simulink model "RCAMSimulation"  (R2024a)
settings: Solver=VariableStepAuto  StartTime=0.0  StopTime=300  RelTol=1e-3
values from neighbouring files (symbols this model uses):
  dt = 1/50    (= 0.02)    [InitializeConstants.m]
  h0 = 250    [InitializeConstants.m]    (also in getDensityParams.m = 0)
  lat0 = deg2rad(47.608013)    [InitializeConstants.m]
  lon0 = deg2rad(-122.335167)    [InitializeConstants.m]
  u0_1 = [-6.32224925618250e-08 ... (first row only)    [InitializeConstants.m]
  u0_2 = [-6.32224925618250e-08 ... (first row only)    [InitializeConstants.m]
  x0 = [227.561443788829 ... (first row only)    [InitializeConstants.m]
undefined symbols (not defined in the file or in its folder): RCAM_Model
libraries: aerolibfltsims x2, matrix_library x1, aerolibanimutils x1
settings Model: Creator=athil  LastModifiedBy=athil
settings OptimizationCC: ReuseModelBlockBuffer=off
settings DebuggingCC: UnconnectedInputMsg=warning  UnconnectedOutputMsg=warning  UnconnectedLineMsg=warning
settings ModelReferenceCC: EnableRefExpFcnMdlSchedulingChecks=on
settings RTWCC: GPUComputeCapability=3.5  DLArmComputeVersion=19.05

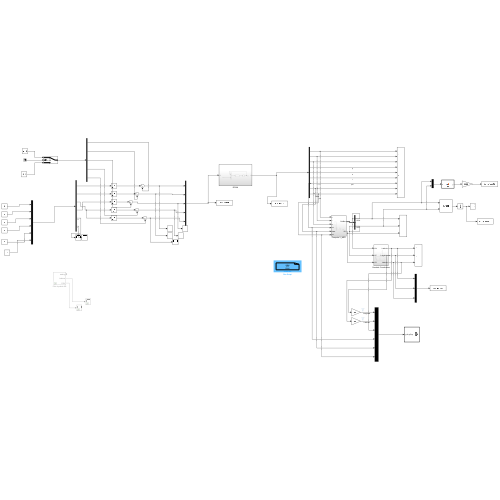
[thumbnail: Simulink's stored preview of the top-level diagram]
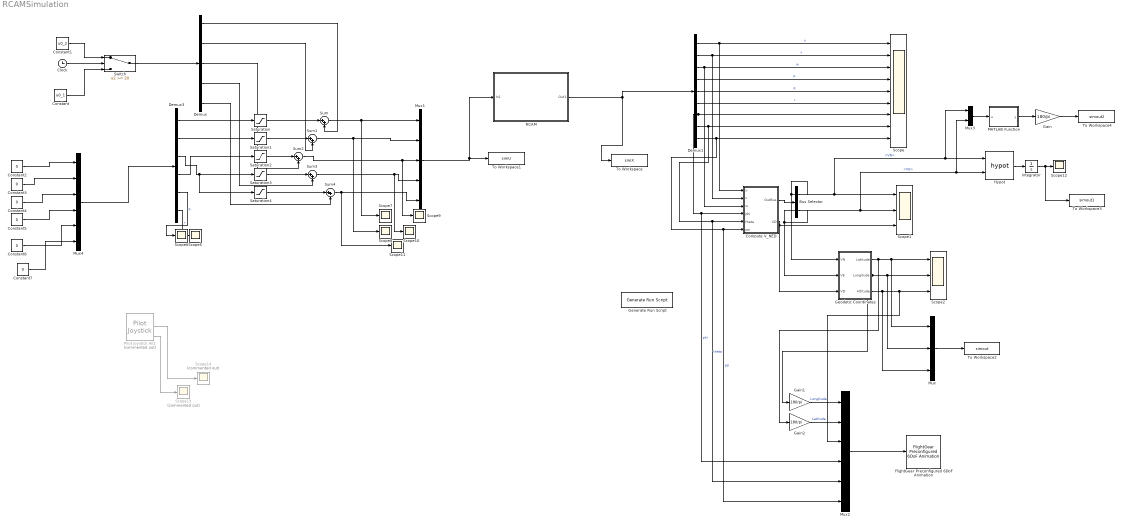
== system RCAMSimulation ==
  Bus Selector : BusSelector  OutputSignals=VN,VE
  Clock : Clock
  Compute V_NED : Subsystem
  Constant : Constant  Value=u0_1
  Constant1 : Constant  Value=u0_2
  Constant{2..7} (6 alike) : Constant  Value=0
  Demux : Demux  Outputs=5
  Demux1 : Demux  Outputs=9
  Demux3 : Demux  Outputs=6
  FlightGear Preconfigured 6DoF Animation : aerolibfltsims/FlightGear Preconfigured 6DoF Animation  xFlightGearVersion=v2019.1  DestinationIpAddress=127.0.0.1  DestinationPort=5502  SampleTime=1/50  packetVersion=24
  Gain : Gain  Gain=180/pi
  Gain1 : Gain  Gain=180/pi
  Gain2 : Gain  Gain=180/pi
  Generate Run Script : aerolibfltsims/Generate Run Script  Architecture=Default  dataFlow=Send  GeometryModelName=767-300  AirportId=KSFO  RunwayId=10L  InitialAltitude=7224  InitialHeading=113  OffsetDistance=4.72  OffsetAzimuth=0  InstallScenery=off  DisableShaders=on  OriginAddress=127.0.0.1  DestinationPort=5502  OriginPort=5505  LocalAddress=127.0.0.1  OutputFileName=runfg.bat  FlightGearBaseDirectory=C:\Program Files\FlightGear 2020.3
  Geodetic Coordinates : Subsystem
  Hypot : Math  Operator=hypot
  Integrator : Integrator
  MATLAB Function : MATLAB Function  TreatAsAtomicUnit=on
  Mux : Mux  Inputs=3
  Mux1 : Mux  Inputs=5
  Mux2 : Mux  Inputs=6
  Mux3 : Mux  Inputs=2
  Mux4 : Mux  Inputs=6
  Pilot Joystick All2 : aerolibanimutils/Pilot Joystick  Commented=on  JoystickID=Joystick1  OutputConfiguration=AllOutputs  SampleTime=dt
  RCAM : Subsystem
  Saturation{,1..4} (5 alike) : Saturate  UpperLimit=0.1  LowerLimit=-0.1
  Scope : Scope  NumInputPorts=9
  Scope1 : Scope  NumInputPorts=3
  Scope{5..12} (8 alike) : Scope
  Scope13 : Scope  Commented=on
  Scope14 : Scope  Commented=on
  Scope2 : Scope  NumInputPorts=3
  Sum{,1..4} (5 alike) : Sum  Inputs=|++
  Switch : Switch  Threshold=20  SaturateOnIntegerOverflow=off  InputSameDT=off
  To Workspace : ToWorkspace  VariableName=simX  SaveFormat=Timeseries  SampleTime=-1
  To Workspace1 : ToWorkspace  VariableName=simU  SaveFormat=Timeseries  SampleTime=-1
  To Workspace2 : ToWorkspace  VariableName=simout  SaveFormat=Timeseries  SampleTime=-1
  To Workspace3 : ToWorkspace  VariableName=simout1  SaveFormat=Timeseries  SampleTime=-1
  To Workspace4 : ToWorkspace  VariableName=simout2  SaveFormat=Timeseries  SampleTime=-1
  wires:
  Demux3/1 -> Saturation/1
  Demux3/2 -> Saturation1/1
  Saturation/1 -> Sum/1
  Mux1/1 -> RCAM/1(In1), To Workspace1/1
  Demux1/1 -> Scope/1, Compute V_NED/1(u)  "u"
  Demux1/3 -> Scope/3, Compute V_NED/3(w)  "w"
  Demux1/4 -> Scope/4  "p"
  Demux1/5 -> Scope/5  "q"
  Demux1/6 -> Scope/6  "r"
  Demux1/7 -> Scope/7, Mux2/4, Compute V_NED/4(phi)  "phi"
  Demux1/8 -> Scope/8, Mux2/5, Compute V_NED/5(theta)  "theta"
  Demux1/9 -> Scope/9, Mux2/6, Compute V_NED/6(psi)  "psi"
  Demux1/2 -> Scope/2, Compute V_NED/2(v)  "v"
  Bus Selector/1 -> Mux3/1, Hypot/1, Scope1/1, Geodetic Coordinates/1(VN)  "<VN>"
  Bus Selector/2 -> Mux3/2, Hypot/2, Scope1/2, Geodetic Coordinates/2(VE)  "<VE>"
  Compute V_NED/2(VD) -> Geodetic Coordinates/3(VD), Scope1/3
  Geodetic Coordinates/1(Latitude) -> Gain2/1, Mux/1, Scope2/1
  Geodetic Coordinates/2(Longitude) -> Gain1/1, Mux/2, Scope2/2
  Mux2/1 -> FlightGear Preconfigured 6DoF Animation/1
  Gain1/1 -> Mux2/1  "Longitude"
  Gain2/1 -> Mux2/2  "Latitude"
  Geodetic Coordinates/3(Altitude) -> Mux/3, Mux2/3, Scope2/3
  RCAM/1(Out1) -> Demux1/1, To Workspace/1
  Demux3/5 -> Scope6/1  "q"
  Demux3/6 -> Scope5/1  "r"
  Mux/1 -> To Workspace2/1
  Compute V_NED/1(OutBus) -> Bus Selector/1
  Demux/1 -> Sum/2
  Sum/1 -> Scope7/1, Mux1/1
  Saturation1/1 -> Sum1/1
  Demux/2 -> Sum1/2
  Sum1/1 -> Scope8/1, Mux1/2
  Saturation2/1 -> Sum2/1
  Demux/3 -> Sum2/2
  Sum2/1 -> Scope9/1, Mux1/3
  Saturation3/1 -> Sum3/1
  Demux/4 -> Sum3/2
  Sum3/1 -> Scope10/1, Mux1/4
  Saturation4/1 -> Sum4/1
  Demux/5 -> Sum4/2
  Sum4/1 -> Scope11/1, Mux1/5
  Demux3/4 -> Saturation2/1
  Demux3/3 -> Saturation4/1, Saturation3/1
  Hypot/1 -> Integrator/1
  Integrator/1 -> To Workspace3/1, Scope12/1
  Mux3/1 -> MATLAB Function/1(u)
  MATLAB Function/1(y) -> Gain/1
  Gain/1 -> To Workspace4/1
  Clock/1 -> Switch/2
  Switch/1 -> Demux/1
  Constant1/1 -> Switch/1
  Constant/1 -> Switch/3
  Pilot Joystick All2/2 -> Scope14/1
  Pilot Joystick All2/3 -> Scope13/1
  Constant2/1 -> Mux4/1
  Constant3/1 -> Mux4/2
  Constant4/1 -> Mux4/3
  Constant5/1 -> Mux4/4
  Constant6/1 -> Mux4/5
  Constant7/1 -> Mux4/6
  Mux4/1 -> Demux3/1

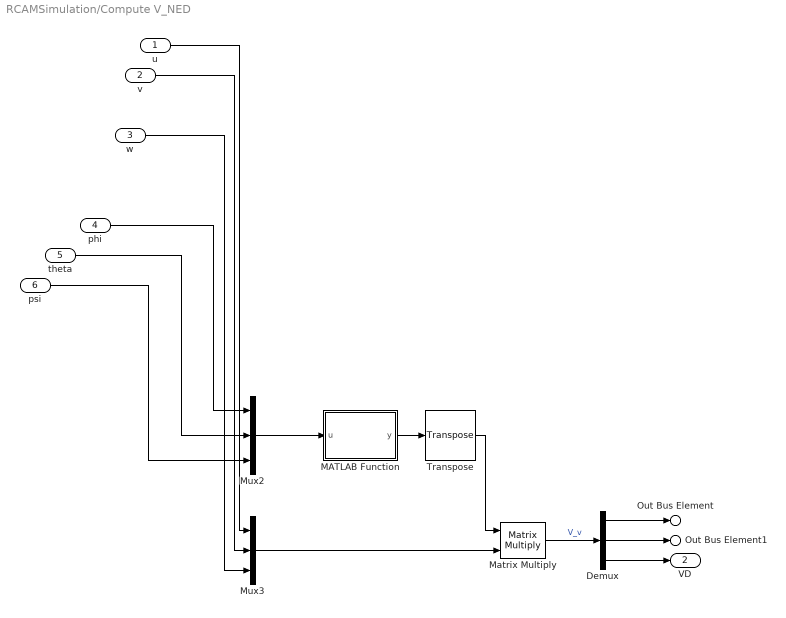
== system RCAMSimulation/Compute V_NED ==
  u : Inport
  v : Inport  Port=2
  w : Inport  Port=3
  phi : Inport  Port=4
  theta : Inport  Port=5
  psi : Inport  Port=6
  Demux : Demux  Outputs=3
  MATLAB Function : MATLAB Function  TreatAsAtomicUnit=on
  Matrix Multiply : Product  Multiplication=Matrix(*)
  Mux2 : Mux  Inputs=3
  Mux3 : Mux  Inputs=3
  Transpose : matrix_library/Transpose
  Out Bus Element : Outport  PortName=OutBus  Element=VN
  Out Bus Element1 : Outport  PortName=OutBus  Element=VE
  VD : Outport  Port=2
  wires:
  MATLAB Function/1(y) -> Transpose/1
  phi/1 -> Mux2/1
  Mux3/1 -> Matrix Multiply/2
  Mux2/1 -> MATLAB Function/1(u)
  Transpose/1 -> Matrix Multiply/1
  v/1 -> Mux3/2
  theta/1 -> Mux2/2
  w/1 -> Mux3/3
  psi/1 -> Mux2/3
  u/1 -> Mux3/1
  Matrix Multiply/1 -> Demux/1  "V_v"
  Demux/1 -> Out Bus Element/1
  Demux/2 -> Out Bus Element1/1
  Demux/3 -> VD/1

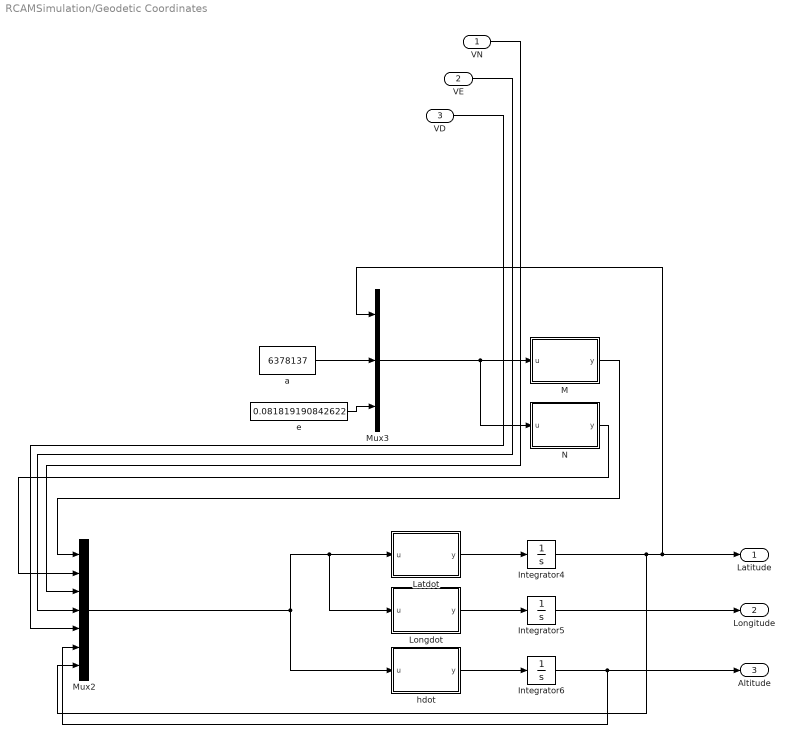
== system RCAMSimulation/Geodetic Coordinates ==
  VN : Inport
  VE : Inport  Port=2
  VD : Inport  Port=3
  Integrator4 : Integrator  InitialCondition=lat0
  Integrator5 : Integrator  InitialCondition=lon0
  Integrator6 : Integrator  InitialCondition=h0
  Latdot : MATLAB Function  TreatAsAtomicUnit=on
  Longdot : MATLAB Function  TreatAsAtomicUnit=on
  M : MATLAB Function  TreatAsAtomicUnit=on
  Mux2 : Mux  Inputs=7
  Mux3 : Mux  Inputs=3
  N : MATLAB Function  TreatAsAtomicUnit=on
  a : Constant  Value=6378137
  e : Constant  Value=0.081819190842622
  hdot : MATLAB Function  TreatAsAtomicUnit=on
  Latitude : Outport
  Longitude : Outport  Port=2
  Altitude : Outport  Port=3
  wires:
  VE/1 -> Mux2/4
  M/1(y) -> Mux2/1
  Integrator6/1 -> Altitude/1, Mux2/6
  hdot/1(y) -> Integrator6/1
  Mux2/1 -> Longdot/1(u), Latdot/1(u), hdot/1(u)
  Mux3/1 -> N/1(u), M/1(u)
  N/1(y) -> Mux2/2
  a/1 -> Mux3/2
  Integrator4/1 -> Mux2/7, Latitude/1, Mux3/1
  e/1 -> Mux3/3
  Latdot/1(y) -> Integrator4/1
  Longdot/1(y) -> Integrator5/1
  Integrator5/1 -> Longitude/1
  VN/1 -> Mux2/3
  VD/1 -> Mux2/5

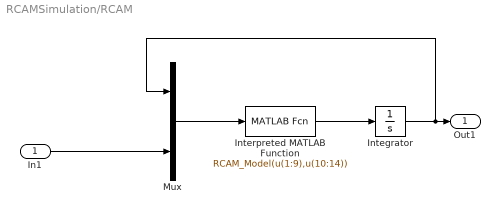
== system RCAMSimulation/RCAM ==
  In1 : Inport
  Integrator : Integrator  InitialCondition=x0
  Interpreted MATLAB Function : MATLABFcn  MATLABFcn=RCAM_Model(u(1:9),u(10:14))
  Mux : Mux  Inputs=2
  Out1 : Outport
  wires:
  Mux/1 -> Interpreted MATLAB Function/1
  In1/1 -> Mux/2
  Interpreted MATLAB Function/1 -> Integrator/1
  Integrator/1 -> Mux/1, Out1/1

== matlab function RCAMSimulation/Compute V_NED/MATLAB Function ==
  data: u input; y output
function y = fcn(u)
phi = u(1);
theta = u(2);
psi = u(3);

C1v = [cos(psi) sin(psi) 0; -sin(psi) cos(psi) 0; 0 0 1];
C21 = [cos(theta) 0 -sin(theta); 0 1 0; sin(theta) 0 cos(theta)];
Cb2 = [1 0 0; 0 cos(phi) sin(phi); 0 -sin(phi) cos(phi)];

y = Cb2 * C21 * C1v;

== matlab function RCAMSimulation/Geodetic Coordinates/N ==
  data: u input; y output
function y = fcn(u)
Latitude = u(1);
a = u(2);
e = u(3);

N = a/ (1 - e^2 * sin(Latitude)^2)^(1/2);
y = N;

== matlab function RCAMSimulation/Geodetic Coordinates/Latdot ==
  data: u input; y output
function y = fcn(u)
M = u(1);
N = u(2);
VN = u(3);
VE = u(4);
VD = u(5);
h = u(6);
Latitude = u(7);

Latdot = VN/(M+h);
y = Latdot;

== matlab function RCAMSimulation/Geodetic Coordinates/Longdot ==
  data: u input; y output
function y = fcn(u)
M = u(1);
N = u(2);
VN = u(3);
VE = u(4);
VD = u(5);
h = u(6);
Latitude = u(7);

Longdot = VE/ ((N + h) * cos(Latitude));
y = Longdot;

== matlab function RCAMSimulation/Geodetic Coordinates/hdot ==
  data: u input; y output
function y = fcn(u)
M = u(1);
N = u(2);
VN = u(3);
VE = u(4);
VD = u(5);
h = u(6);
Latitude = u(7);

hdot = -VD;
y = hdot;

== matlab function RCAMSimulation/MATLAB Function ==
  data: u input; y output
function y = fcn(u)
vN = u(1);
vE = u(2);

z = (3*pi/2)+ mod(atan2(vN,vE),2*pi);
y = 2*pi - z;

== matlab function RCAMSimulation/Geodetic Coordinates/M ==
  data: u input; y output
function y = fcn(u)
Latitude = u(1);
a = u(2);
e = u(3);

M = a * (1  - e^2)/(1 - e^2 * sin(Latitude)^2)^(3/2);
y = M;
